simulink model "top_level"  (R2018a)
settings: Solver=FixedStepAuto  StartTime=0.0  StopTime=inf  FixedStep=0.1  RelTol=1e-3
settings Model: Creator=besho  LastModifiedBy=besho
settings SolverCC: AlgebraicLoopSolver=LineSearch

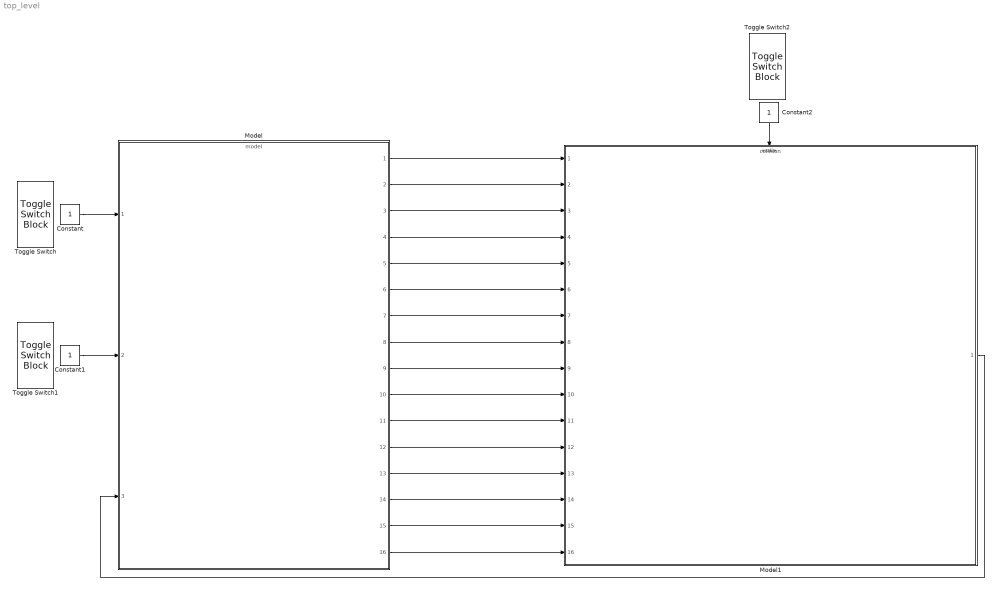
== system top_level ==
  Constant : Constant
  Constant1 : Constant
  Constant2 : Constant
  Model : ModelReference  ModelNameDialog=model.slx  SimulationMode=Normal  ModelReferenceVersion=1.698
  Model1 : ModelReference  ModelNameDialog=collision.slx  SimulationMode=Normal  ModelReferenceVersion=1.107  EnablePortName=Enable  EnablePortStatesWhenEnabling=reset
  Toggle Switch : ToggleSwitchBlock  WebBlockId=3
      settings: Values={{'Off', 'On'}, [0 1]}
  Toggle Switch1 : ToggleSwitchBlock  WebBlockId=4
      settings: Values={{'Off', 'On'}, [0 1]}
  Toggle Switch2 : ToggleSwitchBlock  WebBlockId=7
      settings: Values={{'Off', 'On'}, [0 1]}
  wires:
  Model/1 -> Model1/1
  Model/2 -> Model1/2
  Model/3 -> Model1/3
  Model/4 -> Model1/4
  Model/5 -> Model1/5
  Model/6 -> Model1/6
  Model/7 -> Model1/7
  Model/8 -> Model1/8
  Constant/1 -> Model/1
  Constant1/1 -> Model/2
  Model/9 -> Model1/9
  Model/10 -> Model1/10
  Model/11 -> Model1/11
  Model/12 -> Model1/12
  Model/13 -> Model1/13
  Model/14 -> Model1/14
  Model/15 -> Model1/15
  Model/16 -> Model1/16
  Model1/1 -> Model/3
  Constant2/1 -> Model1/Enable
